simulink model "Sim_Part2_and_3"  (R2017b)
settings: Solver=VariableStepAuto  StartTime=0.0  StopTime=1000  RelTol=1e-3
libraries: simulink x1
settings Model: Creator=Mohammadreza  LastModifiedBy=Mohammadreza

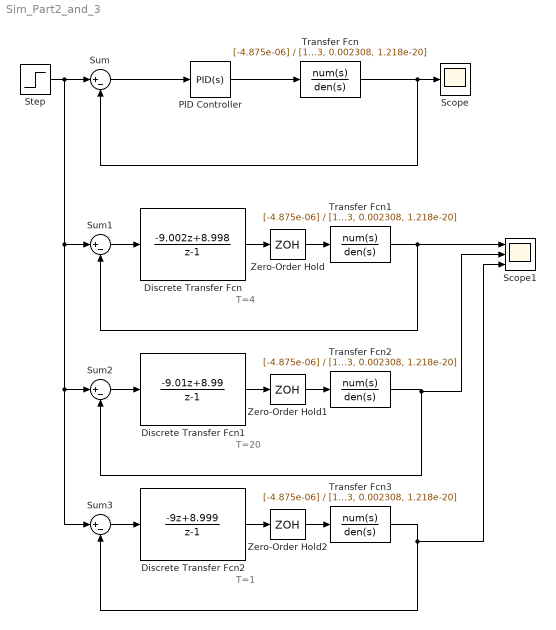
== system Sim_Part2_and_3 ==
  note: T=4
  note: T=20
  note: T=1
  Discrete Transfer Fcn : DiscreteTransferFcn  Numerator=[-9.002 8.998]  Denominator=[1 -1]
  Discrete Transfer Fcn1 : DiscreteTransferFcn  Numerator=[-9.01 8.99]  Denominator=[1 -1]
  Discrete Transfer Fcn2 : DiscreteTransferFcn  Numerator=[-9 8.999]  Denominator=[1 -1]
  PID Controller : simulink/Continuous/PID Controller  Controller=PID  TimeDomain=Continuous-time  SampleTime=-1  IntegratorMethod=Forward Euler  FilterMethod=Forward Euler  Form=Parallel  UseFilter=on  ControllerParametersSource=internal  P=-9  I=-0.001  D=0  N=1000000  InitialConditionSource=internal  InitialConditionForIntegrator=0  InitialConditionForFilter=0  ExternalReset=none  LimitOutput=off  UpperSaturationLimit=inf  LowerSaturationLimit=-inf  LinearizeAsGain=on  AntiWindupMode=none  Kb=1  TrackingMode=off  Kt=1  PParamMin=[]  PParamMax=[]  IParamMin=[]  IParamMax=[]  DParamMin=[]  DParamMax=[]  NParamMin=[]  NParamMax=[]  KbParamMin=[]  KbParamMax=[]  KtParamMin=[]  KtParamMax=[]  POutMin=[]  POutMax=[]  IOutMin=[]  IOutMax=[]  DOutMin=[]  DOutMax=[]  NOutMin=[]  NOutMax=[]  KbOutMin=[]  KbOutMax=[]  KtOutMin=[]  KtOutMax=[]  IntegratorOutMin=[]  IntegratorOutMax=[]  FilterOutMin=[]  FilterOutMax=[]  SumOutMin=[]  SumOutMax=[]  SumI1OutMin=[]  SumI1OutMax=[]  SumI2OutMin=[]  SumI2OutMax=[]  SumI3OutMin=[]  SumI3OutMax=[]  SumDOutMin=[]  SumDOutMax=[]  SaturationOutMin=[]  SaturationOutMax=[]  IntegratorContinuousStateAttributes=''  IntegratorStateMustResolveToSignalObject=off  IntegratorRTWStateStorageClass=Auto  FilterContinuousStateAttributes=''  FilterStateMustResolveToSignalObject=off  FilterRTWStateStorageClass=Auto  DifferentiatorICPrevScaledInput=0  DifferentiatorOutMin=[]  DifferentiatorOutMax=[]  InitialConditionSetting=State (most efficient)  FilterDiffOutCoefMin=[]  FilterDiffOutCoefMax=[]  SumDenOutMin=[]  SumDenOutMax=[]  SumNumOutMin=[]  SumNumOutMax=[]  ReciprocalOutMin=[]  ReciprocalOutMax=[]  DivideOutMin=[]  DivideOutMax=[]  TunerSelectOption=Transfer Function Based (PID Tuner App)
  Scope : Scope
  Scope1 : Scope  NumInputPorts=3
  Step : Step  Time=0  SampleTime=0
  Sum{,1..3} (4 alike) : Sum  Inputs=|+-
  Transfer Fcn{,1..3} (4 alike) : TransferFcn  Numerator=[-4.875e-06]  Denominator=[1, 0.1173, 0.002308, 1.218e-20]
  Zero-Order Hold : ZeroOrderHold  SampleTime=4
  Zero-Order Hold1 : ZeroOrderHold  SampleTime=20
  Zero-Order Hold2 : ZeroOrderHold
  wires:
  Transfer Fcn/1 -> Sum/2, Scope/1
  PID Controller/1 -> Transfer Fcn/1
  Sum/1 -> PID Controller/1
  Transfer Fcn1/1 -> Sum1/2, Scope1/1
  Zero-Order Hold/1 -> Transfer Fcn1/1
  Discrete Transfer Fcn/1 -> Zero-Order Hold/1
  Sum1/1 -> Discrete Transfer Fcn/1
  Transfer Fcn2/1 -> Scope1/2, Sum2/2
  Zero-Order Hold1/1 -> Transfer Fcn2/1
  Zero-Order Hold2/1 -> Transfer Fcn3/1
  Transfer Fcn3/1 -> Scope1/3, Sum3/2
  Step/1 -> Sum3/1, Sum2/1, Sum1/1, Sum/1
  Sum2/1 -> Discrete Transfer Fcn1/1
  Discrete Transfer Fcn1/1 -> Zero-Order Hold1/1
  Discrete Transfer Fcn2/1 -> Zero-Order Hold2/1
  Sum3/1 -> Discrete Transfer Fcn2/1
